simulink library "sensor_failure_lib"  (Simulink 7.2)
settings: Solver=ode45  StartTime=0.0  StopTime=10.0  RelTol=1e-3
undefined symbols (not defined in the file or in its folder): AirData, MAG3, Pots, Vanes
libraries: simulink x24
settings Model: Creator=amurch  LastModifiedBy=gtmdev

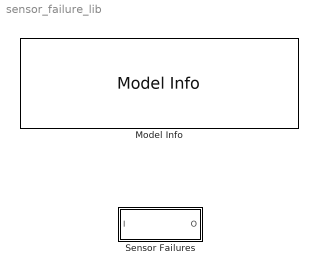
== system sensor_failure_lib ==
  Model Info : simulink/Model-Wide Utilities/Model Info  SystemSampleTime=-1  InitialBlockCM=None  BlockCM=None  Frame=on  DisplayStringWithTags=|  HorizontalTextAlignment=Center  LeftAlignmentValue=0.5  SourceBlockDiagram=sensor_failure_lib  TagMaxNumber=20
      | Sensor Failure Library
      | %<ModelVersion>
      | Las modified by %<LastModifiedBy> on %<LastModificationDate>
  Sensor Failures : Subsystem

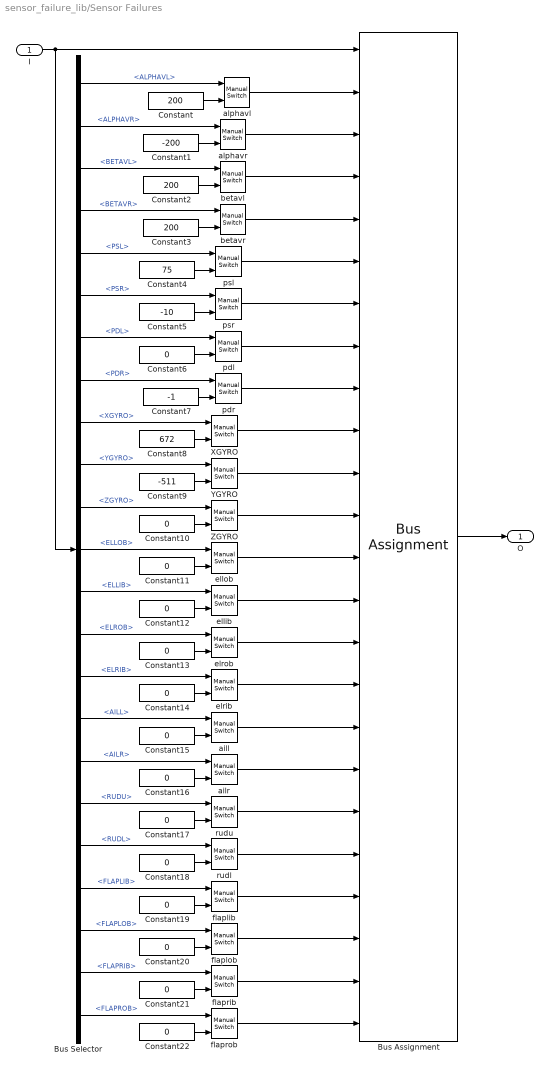
== system sensor_failure_lib/Sensor Failures ==
  I : Inport  OutDataType=sfix(16)  OutScaling=2^0
  Bus Assignment : BusAssignment  AssignedSignals=Vanes.ALPHAVL,Vanes.ALPHAVR,Vanes.BETAVL,Vanes.BETAVR,AirData.PSL,AirData.PSR,AirData.PDL,AirData.PDR,MAG3.XGYRO,MAG3.YGYRO,MAG3.ZGYRO,Pots.ELLOB,Pots.ELLIB,Pots.ELROB,Pots.ELRIB,Pots.AILL,Pots.AILR,Pots.RUDU,Pots.RUDL,Pots.FLAPLIB,Pots.FLAPLOB,Pots.FLAPRIB,Pots.FLAPROB
  Bus Selector : BusSelector  OutputSignals=Vanes.ALPHAVL,Vanes.ALPHAVR,Vanes.BETAVL,Vanes.BETAVR,AirData.PSL,AirData.PSR,AirData.PDL,AirData.PDR,MAG3.XGYRO,MAG3.YGYRO,MAG3.ZGYRO,Pots.ELLOB,Pots.ELLIB,Pots.ELROB,Pots.ELRIB,Pots.AILL,Pots.AILR,Pots.RUDU,Pots.RUDL,Pots.FLAPLIB,Pots.FLAPLOB,Pots.FLAPRIB,Pots.FLAPROB
  Constant : Constant  Value=200  OutDataType=sfix(16)  OutScaling=2^0
  Constant1 : Constant  Value=-200  OutDataType=sfix(16)  OutScaling=2^0
  Constant{6,10..22} (14 alike) : Constant  Value=0  OutDataType=sfix(16)  OutScaling=2^0
  Constant2 : Constant  Value=200  OutDataType=sfix(16)  OutScaling=2^0
  Constant3 : Constant  Value=200  OutDataType=sfix(16)  OutScaling=2^0
  Constant4 : Constant  Value=75  OutDataType=sfix(16)  OutScaling=2^0
  Constant5 : Constant  Value=-10  OutDataType=sfix(16)  OutScaling=2^0
  Constant7 : Constant  Value=-1  OutDataType=sfix(16)  OutScaling=2^0
  Constant8 : Constant  Value=672  OutDataType=sfix(16)  OutScaling=2^0
  Constant9 : Constant  Value=-511  OutDataType=sfix(16)  OutScaling=2^0
  XGYRO : simulink/Signal Routing/Manual Switch  SystemSampleTime=-1  sw=1  action=0  varsize=off
  YGYRO : simulink/Signal Routing/Manual Switch  SystemSampleTime=-1  sw=1  action=0  varsize=off
  ZGYRO : simulink/Signal Routing/Manual Switch  SystemSampleTime=-1  sw=1  action=0  varsize=off
  aill : simulink/Signal Routing/Manual Switch  SystemSampleTime=-1  sw=1  action=0  varsize=off
  ailr : simulink/Signal Routing/Manual Switch  SystemSampleTime=-1  sw=1  action=0  varsize=off
  alphavl : simulink/Signal Routing/Manual Switch  SystemSampleTime=-1  sw=1  action=0  varsize=off
  alphavr : simulink/Signal Routing/Manual Switch  SystemSampleTime=-1  sw=1  action=0  varsize=off
  betavl : simulink/Signal Routing/Manual Switch  SystemSampleTime=-1  sw=1  action=0  varsize=off
  betavr : simulink/Signal Routing/Manual Switch  SystemSampleTime=-1  sw=1  action=0  varsize=off
  ellib : simulink/Signal Routing/Manual Switch  SystemSampleTime=-1  sw=1  action=0  varsize=off
  ellob : simulink/Signal Routing/Manual Switch  SystemSampleTime=-1  sw=1  action=0  varsize=off
  elrib : simulink/Signal Routing/Manual Switch  SystemSampleTime=-1  sw=1  action=0  varsize=off
  elrob : simulink/Signal Routing/Manual Switch  SystemSampleTime=-1  sw=1  action=0  varsize=off
  flaplib : simulink/Signal Routing/Manual Switch  SystemSampleTime=-1  sw=1  action=0  varsize=off
  flaplob : simulink/Signal Routing/Manual Switch  SystemSampleTime=-1  sw=1  action=0  varsize=off
  flaprib : simulink/Signal Routing/Manual Switch  SystemSampleTime=-1  sw=1  action=0  varsize=off
  flaprob : simulink/Signal Routing/Manual Switch  SystemSampleTime=-1  sw=1  action=0  varsize=off
  pdl : simulink/Signal Routing/Manual Switch  SystemSampleTime=-1  sw=1  action=0  varsize=off
  pdr : simulink/Signal Routing/Manual Switch  SystemSampleTime=-1  sw=1  action=0  varsize=off
  psl : simulink/Signal Routing/Manual Switch  SystemSampleTime=-1  sw=1  action=0  varsize=off
  psr : simulink/Signal Routing/Manual Switch  SystemSampleTime=-1  sw=1  action=0  varsize=off
  rudl : simulink/Signal Routing/Manual Switch  SystemSampleTime=-1  sw=1  action=0  varsize=off
  rudu : simulink/Signal Routing/Manual Switch  SystemSampleTime=-1  sw=1  action=0  varsize=off
  O : Outport  OutDataType=sfix(16)  OutScaling=2^0
  wires:
  ZGYRO/1 -> Bus Assignment/12
  Bus Selector/11 -> ZGYRO/1  "<ZGYRO>"
  YGYRO/1 -> Bus Assignment/11
  Bus Selector/10 -> YGYRO/1  "<YGYRO>"
  XGYRO/1 -> Bus Assignment/10
  Bus Selector/9 -> XGYRO/1  "<XGYRO>"
  Constant10/1 -> ZGYRO/2
  Constant9/1 -> YGYRO/2
  Constant8/1 -> XGYRO/2
  I/1 -> Bus Assignment/1, Bus Selector/1
  Bus Assignment/1 -> O/1
  Constant/1 -> alphavl/2
  Bus Selector/1 -> alphavl/1  "<ALPHAVL>"
  alphavl/1 -> Bus Assignment/2
  Constant1/1 -> alphavr/2
  Bus Selector/2 -> alphavr/1  "<ALPHAVR>"
  alphavr/1 -> Bus Assignment/3
  Constant2/1 -> betavl/2
  Bus Selector/3 -> betavl/1  "<BETAVL>"
  betavl/1 -> Bus Assignment/4
  Constant3/1 -> betavr/2
  Bus Selector/4 -> betavr/1  "<BETAVR>"
  betavr/1 -> Bus Assignment/5
  Constant4/1 -> psl/2
  Bus Selector/5 -> psl/1  "<PSL>"
  psl/1 -> Bus Assignment/6
  Constant5/1 -> psr/2
  Bus Selector/6 -> psr/1  "<PSR>"
  psr/1 -> Bus Assignment/7
  Constant6/1 -> pdl/2
  Bus Selector/7 -> pdl/1  "<PDL>"
  pdl/1 -> Bus Assignment/8
  Constant7/1 -> pdr/2
  Bus Selector/8 -> pdr/1  "<PDR>"
  pdr/1 -> Bus Assignment/9
  Bus Selector/12 -> ellob/1  "<ELLOB>"
  Constant11/1 -> ellob/2
  ellob/1 -> Bus Assignment/13
  ellib/1 -> Bus Assignment/14
  elrob/1 -> Bus Assignment/15
  elrib/1 -> Bus Assignment/16
  aill/1 -> Bus Assignment/17
  ailr/1 -> Bus Assignment/18
  rudu/1 -> Bus Assignment/19
  rudl/1 -> Bus Assignment/20
  flaplib/1 -> Bus Assignment/21
  flaplob/1 -> Bus Assignment/22
  flaprib/1 -> Bus Assignment/23
  Bus Selector/13 -> ellib/1  "<ELLIB>"
  Bus Selector/14 -> elrob/1  "<ELROB>"
  Bus Selector/15 -> elrib/1  "<ELRIB>"
  Bus Selector/16 -> aill/1  "<AILL>"
  Bus Selector/17 -> ailr/1  "<AILR>"
  Bus Selector/18 -> rudu/1  "<RUDU>"
  Bus Selector/19 -> rudl/1  "<RUDL>"
  Bus Selector/20 -> flaplib/1  "<FLAPLIB>"
  Bus Selector/21 -> flaplob/1  "<FLAPLOB>"
  Bus Selector/22 -> flaprib/1  "<FLAPRIB>"
  Bus Selector/23 -> flaprob/1  "<FLAPROB>"
  Constant14/1 -> elrib/2
  Constant13/1 -> elrob/2
  Constant12/1 -> ellib/2
  Constant15/1 -> aill/2
  Constant16/1 -> ailr/2
  Constant17/1 -> rudu/2
  Constant18/1 -> rudl/2
  Constant19/1 -> flaplib/2
  Constant20/1 -> flaplob/2
  Constant21/1 -> flaprib/2
  Constant22/1 -> flaprob/2
  flaprob/1 -> Bus Assignment/24
